simulink subsystem "tire_model"  (R2025b)
settings: Solver=VariableStepAuto  StartTime=0.0  StopTime=10.0  RelTol=1e-3
libraries: vehdynlibtire x3, vehdynlibtirecommon x3
settings Model: Creator=jessi  LastModifiedBy=jessi

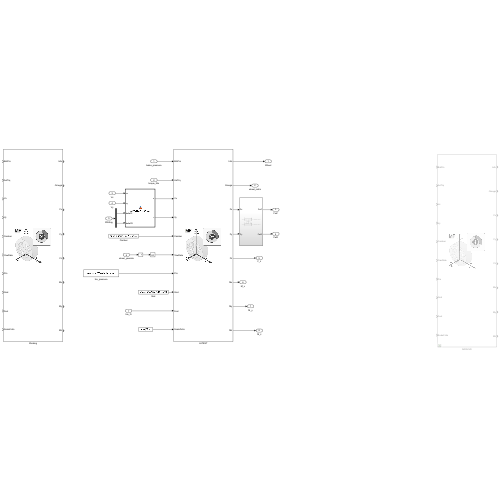
[thumbnail: Simulink's stored preview of the top-level diagram]
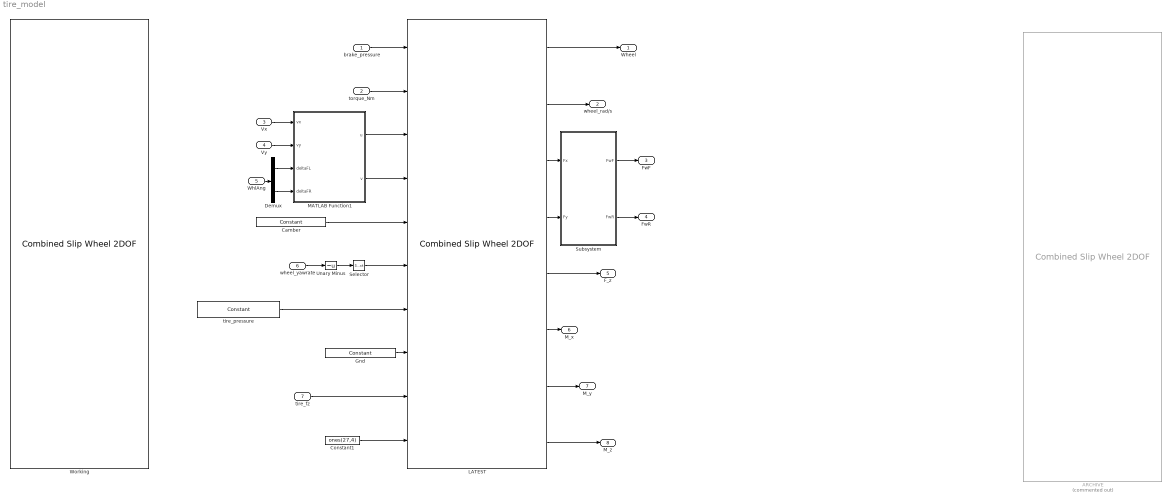
== system tire_model ==
  brake_pressure : Inport  Unit=Pa  PortDimensions=4
  torque_Nm : Inport  Port=2  Unit=N*m  PortDimensions=4
  Vx : Inport  Port=3  Unit=m/s  PortDimensions=4
  Vy : Inport  Port=4  Unit=m/s  PortDimensions=4
  WhlAng : Inport  Port=5
  wheel_yawrate : Inport  Port=6  Unit=rad/s  PortDimensions=1
  tire_fz : Inport  Port=7  Unit=N  PortDimensions=4
  ARCHIVE : vehdynlibtire/Combined Slip Wheel 2DOF  Commented=on  tireType=External file  tireParamSet=C:\Users\jessi\Documents\School\fsae\sim\Hoosier_R25B_B1464_MF.tir  vertType=None  plySteer=off  turnslip=off  BrakeType=Disc  mu_static=.3  mu_kinetic=.2  drum_abore=0.0508  drum_a=0.123  drum_c=0.212  drum_r=0.15  drum_theta1=0  drum_theta2=126  disk_abore=.05  Rm=.177  num_pads=4  brake_p_bpt=[1 11.4736842105263 21.9473684210526 32.4210526315789 42.8947368421053 53.3684210526316 63.8421052631579 74.3157894736842 84.7894736842105 95.2631578947368 105.736842105263 116.210526315789 126.684210526316 137.157894736842 147.631578947368 158.105263157895 168.578947368421 179.052631578947 189.526315789474 200]  brake_n_bpt=[0 52.6315789473684 105.263157894737 157.894736842105 210.526315789474 263.157894736842 315.789473684211 368.421052631579 421.052631578947 473.684210526316 526.315789473684 578.947368421053 631.578947368421 684.210526315789 736.842105263158 789.473684210526 842.105263157895 894.736842105263 947.368421052632 1000]  f_brake_t=[43.4900602404453 42.5056030554862 41.5350898940194 40.5780454442085 39.6340111501808 38.7025443887544 37.7832176914519 36.8756180088306 35.9793460143796 35.0940154454303 34.2192524787115 33.3546951383474 32.4999927342521 31.6548053290159 30.8188032315107 29.991666515561 29.1730845621415 28.362755623661 27.5603864089927 26.765691687993;498.991217495636 487.695866636631 476.560505099801 465.579679307235 454.748127933653 444.060772460445 433.51270824929 423.099196101319 412.81565427025 402.657650900201 392.620896861006 382.701238955775 372.894653477208 363.197240090814 353.605216024701 344.114910546964 334.722759712992 325.425301366216 316.219170376863 307.10109410434;954.492374750826 932.886130217776 911.585920305583 890.581313170261 869.862244717126 849.419000532136 829.242198807128 809.322774193808 789.651962526121 770.221286354971 751.0225412433 732.047782773203 713.289314220164 694.739674852612 676.391628817892 658.238154578366 640.272434863842 622.48784710877 604.877954344734 587.436496520688;1409.99353200602 1378.07639379892 1346.61133551136 1315.58294703329 1284.9763615006 1254.77722860383 1224.97168936497 1195.5463522863 1166.48827078199 1137.78492180974 1109.42418562559 1081.39432659063 1053.68397496312 1026.28210961441 999.178041611083 972.361398609768 945.822110014692 919.550392851325 893.536738312604 867.771898937035;1865.49468926121 1823.26665738007 1781.63675071715 1740.58458089631 1700.09047828407 1660.13545667552 1620.7011799228 1581.76993037878 1543.32457903786 1505.34855726451 1467.82583000789 1430.74087040806 1394.07863570608 1357.82454437621 1321.96445440427 1286.48464264117 1251.37178516554 1216.61293859388 1182.19552228048 1148.10730135338;2320.9958465164 2268.45692096121 2216.66216592293 2165.58621475934 2115.20459506754 2065.49368474721 2016.43067048064 1967.99350847127 1920.16088729373 1872.91219271928 1826.22747439018 1780.08741422549 1734.47329644903 1689.36697913801 1644.75086719747 1600.60788667257 1556.92146031639 1513.67548433643 1470.85430624835 1428.44270376973;2776.49700377159 2713.64718454235 2651.68758112871 2590.58784862237 2530.31871185102 2470.8519128189 2412.16016103848 2354.21708656376 2296.9971955496 2240.47582817405 2184.62911877248 2129.43395804292 2074.86795719199 2020.9094138998 1967.53727999066 1914.73113070398 1862.47113546724 1810.73803007899 1759.51309021622 1708.77810618608;3231.99816102678 3158.8374481235 3086.71299633449 3015.58948248539 2945.43282863449 2876.21014089059 2807.88965159632 2740.44066465625 2673.83350380547 2608.03946362882 2543.03076315477 2478.78050186034 2415.26261793494 2352.4518486616 2290.32369278385 2228.85437473538 2168.02081061809 2107.80057582154 2048.17187418409 1989.11350860242;3687.49931828197 3604.02771170464 3521.73841154027 3440.59111634842 3360.54694541796 3281.56836896228 3203.61914215416 3126.66424274874 3050.66981206134 2975.60309908359 2901.43240753707 2828.12704567777 2755.6572786779 2683.9942834234 2613.11010557704 2542.97761876678 2473.57048576894 2404.8631215641 2336.83065815196 2269.44891101877;4143.00047553716 4049.21797528579 3956.76382674606 3865.59275021144 3775.66106220143 3686.92659703397 3599.34863271199 3512.88782084123 3427.50612031721 3343.16673453836 3259.83405191936 3177.4735894952 3096.05193942085 3015.5367181852 2935.89651837023 2857.10086279818 2779.12016091979 2701.92566730665 2625.48944211983 2549.78431343512;4598.50163279235 4494.40823886693 4391.78924195184 4290.59438407447 4190.77517898491 4092.28482510566 3995.07812326983 3899.11139893372 3804.34242857308 3710.73036999313 3618.23569630166 3526.82013331263 3436.44660016381 3347.079152947 3258.68293116342 3171.22410682959 3084.66983607064 2998.98821304921 2914.1482260877 2830.11971585147;5054.00279004754 4939.59850244808 4826.81465715762 4715.59601793749 4605.88929576838 4497.64305317735 4390.80761382767 4285.3349770262 4181.17873682896 4078.2940054479 3976.63734068395 3876.16667713006 3776.84126090677 3678.62158770879 3581.46934395661 3485.34735086099 ...(+2764 chars)]  NOMPRES=82737.12  PRESMAX=103421  PRESMIN=55158.1  FNOMIN=890.0  FZMAX=3000  FZMIN=100  VXLOW=1  KPUMAX=10  KPUMIN=-1.0  ALPMAX=pi/2  ALPMIN=-pi/2  CAMMAX=0.08726  CAMMIN=-0.08726  LONGVL=11.1  FxRelFreqLwrLim=200*pi  FyRelFreqLwrLim=200*pi  MyRelFreqLwrLim=100*pi  omegao=0  UNLOADED_RADIUS=0.2286  WIDTH=0.1524  RIM_RADIUS=0.127  ASPECT_RATIO=0.67  MASS=9.3  IYY=0.736  br=1e-3  GRAVITY=-9.81  zo=0  zdoto=0  BREFF=0  DREFF=0  FREFF=0  Q_RE0=0  Q_V1=0  Q_V2=0  Q_FZ1=0  Q_FZ2=0  Q_FZ3=0  Q_FCX=0  Q_FCY=0  Q_FCY2=0  PFZ1=0  VERTICAL_STIFFNESS=1  VERTICAL_DAMPING=50  BOTTOM_OFFST=0.01  BOTTOM_STIFF=2000000  Q_CAM1=0  Q_CAM2=0  Q_CAM3=0  Q_FYS1=0  Q_FYS2=0  Q_FYS3=0  LONGITUDINAL_STIFFNESS=183029.97990255515  LATERAL_STIFFNESS=122019.98660170344  PCFX1=6.150634629310016e-19  PCFX2=-0.11842526551903122  PCFX3=0.9999999999999716  PCFY1=6.150634629310016e-19  PCFY2=-0.11842526551903122  PCFY3=0.9999999999999716  Q_RA1=0.671  Q_RA2=0.733  Q_RB1=1.059  Q_RB2=-1.1878  PCX1=1.4779238369371919  PDX1=1.4176795080427544  PDX2=0.07001659216024461  PDX3=4.097157624686553  PEX1=0.24999999999999986  PEX2=-0.4935998299083556  PEX3=0.062308987383295614  PEX4=0.49999999999999994  PKX1=44.40869215364958  PKX2=-0.11467697610242364  PKX3=0.005123300455879327  PHX1=0.00028611316090635194  PHX2=-0.001728319335508632  PVX1=0.004999999999999999  PVX2=0.00477148979863604  PPX1=5.985592437722123e-20  PPX2=-1.4999999999999998  PPX3=-0.45857497477578263  PPX4=-0.43069292241848617  RBX1=7.480599472060266  RBX2=10.358691627632123  RBX3=29.999999999999996  RCX1=1.399999999995603  REX1=-1.1134570691694545  REX2=-0.5558333477828554  RHX1=-9.999999999999997e-07  QSX1=0.0  QSX2=0.5  QSX3=0.05  QSX4=5.0  QSX5=2.0  QSX6=10.0  QSX7=2.0  QSX8=-0.1  QSX9=0.2  QSX10=0.1  QSX11=3.0  QSX12=0  QSX13=0  QSX14=0  PPMX1=0  PCY1=1.42602462123885  PDY1=1.614684806674477  PDY2=-0.25722924030097466  PDY3=7.484237833543449  PEY1=0.24999999999999997  PEY2=0.17282137868029623  PEY3=-0.49999999999981637  PEY4=-18.0131911906531  PEY5=-9.999999999999998  PKY1=-45.05377213726608  PKY2=1.5000000000000002  PKY3=0.9999999999999999  PKY4=1.563548572387517  PKY5=3.062310459473999  PKY6=-4.139177699968599  PKY7=-1.9999999999999998  PHY1=0.002300118354012591  PHY2=-0.0004999941457393199  PVY1=0.06561909162085476  PVY2=-0.057323025837172255  PVY3=-0.7841962281838478  PVY4=-0.4511640295193  PPY1=0.305488175568361  PPY2=0.9999999999971584  PPY3=-0.15059677809127878  PPY4=-6.958531294569729e-28  PPY5=-0.9999999999998861  RBY1=29.999999763033266  RBY2=12.284678148399243  RBY3=9.999999999995652e-07  RBY4=74.99999999999999  RCY1=0.9763806187992715  REY1=0.633343419865921  REY2=0.297623336129197  RHY1=9.999999999999997e-07  RHY2=0.0  RVY1=-0.0009999999999999998  RVY2=-0.001999999999997254  RVY3=-0.049999999999999996  RVY4=1.9999999999999998  RVY5=2.499999999999872  RVY6=-10.881663249213343  QSY1=0.01  QSY2=0.0  QSY3=0.0  QSY4=0.0004  QSY5=0.0  QSY6=0.0  QSY7=0.85  QSY8=0.45  QBZ1=6.523760266884923  QBZ2=-1.0654322141006967  QBZ3=0.0  QBZ4=0.0  QBZ5=-1.0  QBZ6=0  QBZ9=6.716054935778435  QBZ10=0.0  QCZ1=1.1  QDZ1=0.1344522977151938  QDZ2=-0.04833102317146014  QDZ3=0.5  QDZ4=-1.5  QDZ6=0.01667575088116158  QDZ7=-0.026005524615869646  QDZ8=-0.5  QDZ9=0.02  QDZ10=0.0  QDZ11=0.0  QEZ1=-6.042645141020775  QEZ2=5.302859320838443  QEZ3=13.524667353097806  QEZ4=0.17736241081250134  QEZ5=-2.0  QHZ1=0.00824419812657765  QHZ2=0.004999999999999817  QHZ3=0.0  QHZ4=0.0  PPZ1=0.5  PPZ2=0.0  SSZ1=0.0  SSZ2=0.0  SSZ3=0.0  SSZ4=0.0  PDXP1=0.4  PDXP2=0  PDXP3=0  PKYP1=1  PDYP1=0.4  PDYP2=0  PDYP3=0  PDYP4=0  PHYP1=1  PHYP2=0.15  PHYP3=0  PHYP4=-4  PECP1=2.5  PECP2=0.0  QDTP1=10  QCRP1=0.2  QCRP2=0.1  QBRP1=0.1  QDRP1=1  QDRP2=0  aMode=2
  Camber : vehdynlibtirecommon/Constant  const=0  numWheels=4
  Constant1 : Constant  Value=ones(27,4)
  Demux : Demux  Outputs=2
  Gnd : vehdynlibtirecommon/Constant  const=0  numWheels=4
  LATEST : vehdynlibtire/Combined Slip Wheel 2DOF  tireType=External file  tireParamSet=C:\Users\jessi\Documents\School\fsae\sim\heiko_tires_2.tir  vertType=None  plySteer=off  turnslip=off  BrakeType=Disc  mu_static=.3  mu_kinetic=.2  drum_abore=0.0508  drum_a=0.123  drum_c=0.212  drum_r=0.15  drum_theta1=0  drum_theta2=126  disk_abore=.05  Rm=.177  num_pads=4  brake_p_bpt=[1 11.4736842105263 21.9473684210526 32.4210526315789 42.8947368421053 53.3684210526316 63.8421052631579 74.3157894736842 84.7894736842105 95.2631578947368 105.736842105263 116.210526315789 126.684210526316 137.157894736842 147.631578947368 158.105263157895 168.578947368421 179.052631578947 189.526315789474 200]  brake_n_bpt=[0 52.6315789473684 105.263157894737 157.894736842105 210.526315789474 263.157894736842 315.789473684211 368.421052631579 421.052631578947 473.684210526316 526.315789473684 578.947368421053 631.578947368421 684.210526315789 736.842105263158 789.473684210526 842.105263157895 894.736842105263 947.368421052632 1000]  f_brake_t=[43.4900602404453 42.5056030554862 41.5350898940194 40.5780454442085 39.6340111501808 38.7025443887544 37.7832176914519 36.8756180088306 35.9793460143796 35.0940154454303 34.2192524787115 33.3546951383474 32.4999927342521 31.6548053290159 30.8188032315107 29.991666515561 29.1730845621415 28.362755623661 27.5603864089927 26.765691687993;498.991217495636 487.695866636631 476.560505099801 465.579679307235 454.748127933653 444.060772460445 433.51270824929 423.099196101319 412.81565427025 402.657650900201 392.620896861006 382.701238955775 372.894653477208 363.197240090814 353.605216024701 344.114910546964 334.722759712992 325.425301366216 316.219170376863 307.10109410434;954.492374750826 932.886130217776 911.585920305583 890.581313170261 869.862244717126 849.419000532136 829.242198807128 809.322774193808 789.651962526121 770.221286354971 751.0225412433 732.047782773203 713.289314220164 694.739674852612 676.391628817892 658.238154578366 640.272434863842 622.48784710877 604.877954344734 587.436496520688;1409.99353200602 1378.07639379892 1346.61133551136 1315.58294703329 1284.9763615006 1254.77722860383 1224.97168936497 1195.5463522863 1166.48827078199 1137.78492180974 1109.42418562559 1081.39432659063 1053.68397496312 1026.28210961441 999.178041611083 972.361398609768 945.822110014692 919.550392851325 893.536738312604 867.771898937035;1865.49468926121 1823.26665738007 1781.63675071715 1740.58458089631 1700.09047828407 1660.13545667552 1620.7011799228 1581.76993037878 1543.32457903786 1505.34855726451 1467.82583000789 1430.74087040806 1394.07863570608 1357.82454437621 1321.96445440427 1286.48464264117 1251.37178516554 1216.61293859388 1182.19552228048 1148.10730135338;2320.9958465164 2268.45692096121 2216.66216592293 2165.58621475934 2115.20459506754 2065.49368474721 2016.43067048064 1967.99350847127 1920.16088729373 1872.91219271928 1826.22747439018 1780.08741422549 1734.47329644903 1689.36697913801 1644.75086719747 1600.60788667257 1556.92146031639 1513.67548433643 1470.85430624835 1428.44270376973;2776.49700377159 2713.64718454235 2651.68758112871 2590.58784862237 2530.31871185102 2470.8519128189 2412.16016103848 2354.21708656376 2296.9971955496 2240.47582817405 2184.62911877248 2129.43395804292 2074.86795719199 2020.9094138998 1967.53727999066 1914.73113070398 1862.47113546724 1810.73803007899 1759.51309021622 1708.77810618608;3231.99816102678 3158.8374481235 3086.71299633449 3015.58948248539 2945.43282863449 2876.21014089059 2807.88965159632 2740.44066465625 2673.83350380547 2608.03946362882 2543.03076315477 2478.78050186034 2415.26261793494 2352.4518486616 2290.32369278385 2228.85437473538 2168.02081061809 2107.80057582154 2048.17187418409 1989.11350860242;3687.49931828197 3604.02771170464 3521.73841154027 3440.59111634842 3360.54694541796 3281.56836896228 3203.61914215416 3126.66424274874 3050.66981206134 2975.60309908359 2901.43240753707 2828.12704567777 2755.6572786779 2683.9942834234 2613.11010557704 2542.97761876678 2473.57048576894 2404.8631215641 2336.83065815196 2269.44891101877;4143.00047553716 4049.21797528579 3956.76382674606 3865.59275021144 3775.66106220143 3686.92659703397 3599.34863271199 3512.88782084123 3427.50612031721 3343.16673453836 3259.83405191936 3177.4735894952 3096.05193942085 3015.5367181852 2935.89651837023 2857.10086279818 2779.12016091979 2701.92566730665 2625.48944211983 2549.78431343512;4598.50163279235 4494.40823886693 4391.78924195184 4290.59438407447 4190.77517898491 4092.28482510566 3995.07812326983 3899.11139893372 3804.34242857308 3710.73036999313 3618.23569630166 3526.82013331263 3436.44660016381 3347.079152947 3258.68293116342 3171.22410682959 3084.66983607064 2998.98821304921 2914.1482260877 2830.11971585147;5054.00279004754 4939.59850244808 4826.81465715762 4715.59601793749 4605.88929576838 4497.64305317735 4390.80761382767 4285.3349770262 4181.17873682896 4078.2940054479 3976.63734068395 3876.16667713006 3776.84126090677 3678.62158770879 3581.46934395661 3485.34735086099 ...(+2764 chars)]  NOMPRES=82737.12  PRESMAX=103421  PRESMIN=55158.1  FNOMIN=890  FZMAX=2500  FZMIN=100  VXLOW=1  KPUMAX=10  KPUMIN=-1  ALPMAX=1.5708  ALPMIN=-1.5708  CAMMAX=0.08726  CAMMIN=-0.08726  LONGVL=11.1  FxRelFreqLwrLim=200*pi  FyRelFreqLwrLim=200*pi  MyRelFreqLwrLim=100*pi  omegao=0  UNLOADED_RADIUS=0.2286  WIDTH=0.1524  RIM_RADIUS=0.127  ASPECT_RATIO=0.67  MASS=9.3  IYY=0.736  br=1e-3  GRAVITY=-9.81  zo=0  zdoto=0  BREFF=8.386  DREFF=0.25826  FREFF=0.07394  Q_RE0=0.9974  Q_V1=0.00077  Q_V2=0.04667  Q_FZ1=0  Q_FZ2=15.4  Q_FZ3=0  Q_FCX=0  Q_FCY=0  Q_FCY2=0  PFZ1=0.7098  VERTICAL_STIFFNESS=209651  VERTICAL_DAMPING=50  BOTTOM_OFFST=0.01  BOTTOM_STIFF=2000000  Q_CAM1=0  Q_CAM2=0  Q_CAM3=0  Q_FYS1=0  Q_FYS2=0  Q_FYS3=0  LONGITUDINAL_STIFFNESS=180205.884260107  LATERAL_STIFFNESS=120137.256173405  PCFX1=4.99782632605843e-29  PCFX2=0.0455980345994856  PCFX3=1  PCFY1=4.99782632605843e-29  PCFY2=0.0455980345994856  PCFY3=1  Q_RA1=0.671  Q_RA2=0.733  Q_RB1=1.059  Q_RB2=-1.1878  PCX1=1.47792  PDX1=1.41768  PDX2=0.0700166  PDX3=4.09716  PEX1=0.25  PEX2=-0.4936  PEX3=0.062309  PEX4=0.5  PKX1=44.4087  PKX2=-0.114677  PKX3=0.0051233  PHX1=0.000286113  PHX2=-0.00172832  PVX1=0.005  PVX2=0.00477149  PPX1=5.9855924377e-20  PPX2=-1.5  PPX3=-0.458575  PPX4=-0.430693  RBX1=7.4806  RBX2=10.3587  RBX3=30  RCX1=1.4  REX1=-1.11346  REX2=-0.555833  RHX1=-1e-06  QSX1=0  QSX2=0.5  QSX3=0.05  QSX4=5  QSX5=2  QSX6=10  QSX7=2  QSX8=-0.1  QSX9=0.2  QSX10=0.1  QSX11=3  QSX12=0  QSX13=0  QSX14=0  PPMX1=0  PCY1=1.1204  PDY1=1.64222  PDY2=-0.32532  PDY3=8.96121  PEY1=-0.353569  PEY2=0.5  PEY3=0.5  PEY4=-4.334674291e-12  PEY5=-10  PKY1=-58.8756  PKY2=2.6  PKY3=0.82447  PKY4=1.73528  PKY5=0.246779  PKY6=-4.06378  PKY7=-2  PHY1=0.00182546  PHY2=0.000636193  PVY1=0.05  PVY2=-0.0036552  PVY3=0.0983321  PVY4=0.0465855  PPY1=0.569312  PPY2=1  PPY3=-0.151827  PPY4=-1.6963735362e-22  PPY5=-1  RBY1=29.9998  RBY2=12.134  RBY3=9.9999999999e-07  RBY4=75  RCY1=0.965142  REY1=0.61543  REY2=0.174596  RHY1=1e-06  RHY2=0  RVY1=-0.001  RVY2=-0.002  RVY3=-0.05  RVY4=-2  RVY5=2.5  RVY6=-11.3254  QSY1=0.01  QSY2=0  QSY3=0  QSY4=0.0004  QSY5=0  QSY6=0  QSY7=0.85  QSY8=0.45  QBZ1=6.60806  QBZ2=-1.78557  QBZ3=0  QBZ4=0  QBZ5=-1  QBZ6=0  QBZ9=6.54673  QBZ10=0  QCZ1=1.1  QDZ1=0.136052  QDZ2=-0.0673485  QDZ3=0.5  QDZ4=-1.5  QDZ6=0.0171131  QDZ7=-0.028301  QDZ8=-0.5  QDZ9=0.02  QDZ10=0  QDZ11=0  QEZ1=-5.88202  QEZ2=4.83736  QEZ3=13.7151  QEZ4=0.191406  QEZ5=-2  QHZ1=0.00841306  QHZ2=0.005  QHZ3=0  QHZ4=0  PPZ1=0.5  PPZ2=0  SSZ1=0  SSZ2=0  SSZ3=0  SSZ4=0  PDXP1=0.4  PDXP2=0  PDXP3=0  PKYP1=1  PDYP1=0.4  PDYP2=0  PDYP3=0  PDYP4=0  PHYP1=1  PHYP2=0.15  PHYP3=0  PHYP4=-4  PECP1=0.5  PECP2=0  QDTP1=10  QCRP1=0.2  QCRP2=0.1  QBRP1=0.1  QDRP1=1  QDRP2=0  aMode=2
  MATLAB Function1 : MATLAB Function  TreatAsAtomicUnit=on
  Selector : Selector  InputPortWidth=1  IndexOptions=Index vector (dialog)  Indices=[1 1 1 1]  OutputSizes=1
  Subsystem : Subsystem
  Unary Minus : UnaryMinus
  Working : vehdynlibtire/Combined Slip Wheel 2DOF  tireType=External file  vertType=None  plySteer=off  turnslip=off  BrakeType=Disc  mu_static=.3  mu_kinetic=.2  drum_abore=0.0508  drum_a=0.123  drum_c=0.212  drum_r=0.15  drum_theta1=0  drum_theta2=126  disk_abore=.05  Rm=.177  num_pads=4  brake_p_bpt=[1 11.4736842105263 21.9473684210526 32.4210526315789 42.8947368421053 53.3684210526316 63.8421052631579 74.3157894736842 84.7894736842105 95.2631578947368 105.736842105263 116.210526315789 126.684210526316 137.157894736842 147.631578947368 158.105263157895 168.578947368421 179.052631578947 189.526315789474 200]  brake_n_bpt=[0 52.6315789473684 105.263157894737 157.894736842105 210.526315789474 263.157894736842 315.789473684211 368.421052631579 421.052631578947 473.684210526316 526.315789473684 578.947368421053 631.578947368421 684.210526315789 736.842105263158 789.473684210526 842.105263157895 894.736842105263 947.368421052632 1000]  f_brake_t=[43.4900602404453 42.5056030554862 41.5350898940194 40.5780454442085 39.6340111501808 38.7025443887544 37.7832176914519 36.8756180088306 35.9793460143796 35.0940154454303 34.2192524787115 33.3546951383474 32.4999927342521 31.6548053290159 30.8188032315107 29.991666515561 29.1730845621415 28.362755623661 27.5603864089927 26.765691687993;498.991217495636 487.695866636631 476.560505099801 465.579679307235 454.748127933653 444.060772460445 433.51270824929 423.099196101319 412.81565427025 402.657650900201 392.620896861006 382.701238955775 372.894653477208 363.197240090814 353.605216024701 344.114910546964 334.722759712992 325.425301366216 316.219170376863 307.10109410434;954.492374750826 932.886130217776 911.585920305583 890.581313170261 869.862244717126 849.419000532136 829.242198807128 809.322774193808 789.651962526121 770.221286354971 751.0225412433 732.047782773203 713.289314220164 694.739674852612 676.391628817892 658.238154578366 640.272434863842 622.48784710877 604.877954344734 587.436496520688;1409.99353200602 1378.07639379892 1346.61133551136 1315.58294703329 1284.9763615006 1254.77722860383 1224.97168936497 1195.5463522863 1166.48827078199 1137.78492180974 1109.42418562559 1081.39432659063 1053.68397496312 1026.28210961441 999.178041611083 972.361398609768 945.822110014692 919.550392851325 893.536738312604 867.771898937035;1865.49468926121 1823.26665738007 1781.63675071715 1740.58458089631 1700.09047828407 1660.13545667552 1620.7011799228 1581.76993037878 1543.32457903786 1505.34855726451 1467.82583000789 1430.74087040806 1394.07863570608 1357.82454437621 1321.96445440427 1286.48464264117 1251.37178516554 1216.61293859388 1182.19552228048 1148.10730135338;2320.9958465164 2268.45692096121 2216.66216592293 2165.58621475934 2115.20459506754 2065.49368474721 2016.43067048064 1967.99350847127 1920.16088729373 1872.91219271928 1826.22747439018 1780.08741422549 1734.47329644903 1689.36697913801 1644.75086719747 1600.60788667257 1556.92146031639 1513.67548433643 1470.85430624835 1428.44270376973;2776.49700377159 2713.64718454235 2651.68758112871 2590.58784862237 2530.31871185102 2470.8519128189 2412.16016103848 2354.21708656376 2296.9971955496 2240.47582817405 2184.62911877248 2129.43395804292 2074.86795719199 2020.9094138998 1967.53727999066 1914.73113070398 1862.47113546724 1810.73803007899 1759.51309021622 1708.77810618608;3231.99816102678 3158.8374481235 3086.71299633449 3015.58948248539 2945.43282863449 2876.21014089059 2807.88965159632 2740.44066465625 2673.83350380547 2608.03946362882 2543.03076315477 2478.78050186034 2415.26261793494 2352.4518486616 2290.32369278385 2228.85437473538 2168.02081061809 2107.80057582154 2048.17187418409 1989.11350860242;3687.49931828197 3604.02771170464 3521.73841154027 3440.59111634842 3360.54694541796 3281.56836896228 3203.61914215416 3126.66424274874 3050.66981206134 2975.60309908359 2901.43240753707 2828.12704567777 2755.6572786779 2683.9942834234 2613.11010557704 2542.97761876678 2473.57048576894 2404.8631215641 2336.83065815196 2269.44891101877;4143.00047553716 4049.21797528579 3956.76382674606 3865.59275021144 3775.66106220143 3686.92659703397 3599.34863271199 3512.88782084123 3427.50612031721 3343.16673453836 3259.83405191936 3177.4735894952 3096.05193942085 3015.5367181852 2935.89651837023 2857.10086279818 2779.12016091979 2701.92566730665 2625.48944211983 2549.78431343512;4598.50163279235 4494.40823886693 4391.78924195184 4290.59438407447 4190.77517898491 4092.28482510566 3995.07812326983 3899.11139893372 3804.34242857308 3710.73036999313 3618.23569630166 3526.82013331263 3436.44660016381 3347.079152947 3258.68293116342 3171.22410682959 3084.66983607064 2998.98821304921 2914.1482260877 2830.11971585147;5054.00279004754 4939.59850244808 4826.81465715762 4715.59601793749 4605.88929576838 4497.64305317735 4390.80761382767 4285.3349770262 4181.17873682896 4078.2940054479 3976.63734068395 3876.16667713006 3776.84126090677 3678.62158770879 3581.46934395661 3485.34735086099 ...(+2764 chars)]  NOMPRES=82737.12  PRESMAX=103421  PRESMIN=55158.1  FNOMIN=890.0  FZMAX=5000  FZMIN=100  VXLOW=1  KPUMAX=10  KPUMIN=-1.0  ALPMAX=pi/2  ALPMIN=-pi/2  CAMMAX=0.08726  CAMMIN=-0.08726  LONGVL=11.1  FxRelFreqLwrLim=200*pi  FyRelFreqLwrLim=200*pi  MyRelFreqLwrLim=100*pi  omegao=0  UNLOADED_RADIUS=0.2286  WIDTH=0.1524  RIM_RADIUS=0.127  ASPECT_RATIO=0.67  MASS=9.3  IYY=0.736  br=1e-3  GRAVITY=-9.81  zo=0  zdoto=0  BREFF=8.386  DREFF=0.25826  FREFF=0.07394  Q_RE0=0.9974  Q_V1=0.00077  Q_V2=0.04667  Q_FZ1=0  Q_FZ2=15.4  Q_FZ3=0  Q_FCX=0  Q_FCY=0  Q_FCY2=0  PFZ1=0.7098  VERTICAL_STIFFNESS=209651  VERTICAL_DAMPING=50  BOTTOM_OFFST=0.01  BOTTOM_STIFF=2000000  Q_CAM1=0  Q_CAM2=0  Q_CAM3=0  Q_FYS1=0  Q_FYS2=0  Q_FYS3=0  LONGITUDINAL_STIFFNESS=358066  LATERAL_STIFFNESS=102673  PCFX1=0.17504  PCFX2=0  PCFX3=0  PCFY1=0.16365  PCFY2=0  PCFY3=0.24993  Q_RA1=0.671  Q_RA2=0.733  Q_RB1=1.059  Q_RB2=-1.1878  PCX1=1.4759319652841167  PDX1=2.1796047139413703  PDX2=-0.4291518578855814  PDX3=9.999999999999998  PEX1=0.24999999999999992  PEX2=0.4999999999503354  PEX3=-0.19999999998013418  PEX4=0.49999999999999994  PKX1=44.486722871854106  PKX2=0.7120674645715347  PKX3=0.05499344672791521  PHX1=0.00028868605457366223  PHX2=0.0019999999988281974  PVX1=0.004999999999999999  PVX2=-0.004999999999999571  PPX1=2.4205061531330237e-17  PPX2=-0.9573016482413841  PPX3=-0.44725115013003364  PPX4=-1.0829178486140199  RBX1=7.492442914324831  RBX2=10.346089331771397  RBX3=29.999999999999996  RCX1=1.3999999999999924  REX1=-1.157802528712476  REX2=0.9999999999999999  RHX1=-9.999999999999997e-07  QSX1=0.0  QSX2=0.5  QSX3=0.05  QSX4=5.0  QSX5=2.0  QSX6=10.0  QSX7=2.0  QSX8=-0.1  QSX9=0.2  QSX10=0.1  QSX11=3.0  QSX12=0  QSX13=0  QSX14=0  PPMX1=0  PCY1=1.4260605641217314  PDY1=2.4841487233120225  PDY2=-0.1876440219775705  PDY3=7.508428290647241  PEY1=0.24999999999999997  PEY2=-0.499999999999991  PEY3=-0.49999999999981753  PEY4=-18.269893351294126  PEY5=9.999999999999998  PKY1=-45.05302401059848  PKY2=2.1781682283379564  PKY3=-0.17604712854342697  PKY4=1.9426288921522195  PKY5=4.999999999999999  PKY6=-4.17394673832909  PKY7=-1.7192793969581321  PHY1=0.0023001682759390277  PHY2=0.0031347378176419653  PVY1=0.06560934751893403  PVY2=0.11060727790094066  PVY3=-0.7870245501487243  PVY4=1.9999999990891213  PPY1=0.15987950056064024  PPY2=0.8091878858639612  PPY3=-0.0679339736908627  PPY4=-0.3106544629486843  PPY5=-0.9999999999987371  RBY1=23.942508490286457  RBY2=10.659317359995574  RBY3=7.459484998984083e-07  RBY4=-74.99999999999963  RCY1=0.9838718951518215  REY1=0.571655288653177  REY2=0.6687626858266051  RHY1=9.99998578319522e-07  RHY2=0.0  RVY1=0.0009999999999997134  RVY2=0.001999999999999887  RVY3=-0.049999999999999996  RVY4=-1.9999999999999998  RVY5=2.4999447302580524  RVY6=9.5344602632312  QSY1=0.01  QSY2=0.0  QSY3=0.0  QSY4=0.0004  QSY5=0.0  QSY6=0.0  QSY7=0.85  QSY8=0.45  QBZ1=10.0  QBZ2=-2.0  QBZ3=0.0  QBZ4=0.0  QBZ5=-1.0  QBZ6=0  QBZ9=15.0  QBZ10=0.0  QCZ1=1.1  QDZ1=0.12  QDZ2=-0.02  QDZ3=0.5  QDZ4=-1.5  QDZ6=-0.01  QDZ7=0.01  QDZ8=-0.5  QDZ9=0.02  QDZ10=0.0  QDZ11=0.0  QEZ1=-1.5  QEZ2=-0.5  QEZ3=0.0  QEZ4=0.2  QEZ5=-2.0  QHZ1=0.005  QHZ2=0.002  QHZ3=0.0  QHZ4=0.0  PPZ1=0.5  PPZ2=0.0  SSZ1=0.0  SSZ2=0.0  SSZ3=0.0  SSZ4=0.0  PDXP1=0.4  PDXP2=0  PDXP3=0  PKYP1=1  PDYP1=0.4  PDYP2=0  PDYP3=0  PDYP4=0  PHYP1=1  PHYP2=0.15  PHYP3=0  PHYP4=-4  PECP1=2.5  PECP2=0.0  QDTP1=10  QCRP1=0.2  QCRP2=0.1  QBRP1=0.1  QDRP1=1  QDRP2=0  aMode=2
  tire_pressure : vehdynlibtirecommon/Constant  const=2.4e5*1.1  numWheels=4
  Wheel : Outport
  wheel_rad/s : Outport  Port=2  Unit=rad/s  PortDimensions=4
  FwF : Outport  Port=3  Unit=N  PortDimensions=[2 2]
  FwR : Outport  Port=4  PortDimensions=[2 2]
  F_z : Outport  Port=5
  M_x : Outport  Port=6
  M_y : Outport  Port=7
  M_z : Outport  Port=8
  wires:
  WhlAng/1 -> Demux/1
  Subsystem/1(FwF) -> FwF/1
  Subsystem/2(FwR) -> FwR/1
  Vx/1 -> MATLAB Function1/1(vx)
  Vy/1 -> MATLAB Function1/2(vy)
  Demux/1 -> MATLAB Function1/3(deltaFL)
  Demux/2 -> MATLAB Function1/4(deltaFR)
  wheel_yawrate/1 -> Unary Minus/1
  Unary Minus/1 -> Selector/1
  tire_fz/1 -> LATEST/9
  LATEST/4 -> Subsystem/2(Fy)
  Gnd/1 -> LATEST/8
  Camber/1 -> LATEST/5
  tire_pressure/1 -> LATEST/7
  torque_Nm/1 -> LATEST/2
  LATEST/2 -> wheel_rad/s/1
  MATLAB Function1/1(u) -> LATEST/3
  LATEST/5 -> F_z/1
  LATEST/6 -> M_x/1
  LATEST/7 -> M_y/1
  LATEST/8 -> M_z/1
  Selector/1 -> LATEST/6
  Constant1/1 -> LATEST/10
  brake_pressure/1 -> LATEST/1
  LATEST/3 -> Subsystem/1(Fx)
  MATLAB Function1/2(v) -> LATEST/4
  LATEST/1 -> Wheel/1

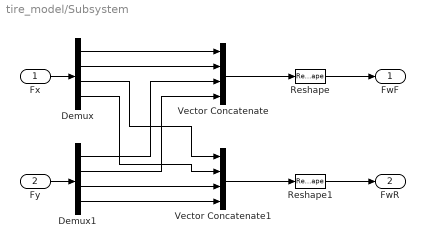
== system tire_model/Subsystem ==
  Fx : Inport
  Fy : Inport  Port=2
  Demux : Demux
  Demux1 : Demux
  Reshape : Reshape  OutputDimensionality=Customize  OutputDimensions=[2,2]
  Reshape1 : Reshape  OutputDimensionality=Customize  OutputDimensions=[2,2]
  Vector Concatenate : Concatenate  NumInputs=4
  Vector Concatenate1 : Concatenate  NumInputs=4
  FwF : Outport
  FwR : Outport  Port=2
  wires:
  Reshape/1 -> FwF/1
  Demux1/2 -> Vector Concatenate/4
  Fx/1 -> Demux/1
  Demux1/4 -> Vector Concatenate1/4
  Demux1/3 -> Vector Concatenate1/3
  Demux1/1 -> Vector Concatenate/3
  Demux/3 -> Vector Concatenate1/1
  Fy/1 -> Demux1/1
  Demux/4 -> Vector Concatenate1/2
  Demux/1 -> Vector Concatenate/1
  Vector Concatenate/1 -> Reshape/1
  Demux/2 -> Vector Concatenate/2
  Vector Concatenate1/1 -> Reshape1/1
  Reshape1/1 -> FwR/1

== matlab function tire_model/MATLAB Function1 ==
  data: vx input; u output; vy input; deltaFL input; deltaFR input; v output
function [u, v] = vehToTireFrontSteer(vx, vy, deltaFL, deltaFR)
%#codegen
u = zeros(4,1);
v = zeros(4,1);

vx = reshape(vx,4,1);
vy = reshape(vy,4,1);

delta = [deltaFL; deltaFR; 0; 0];   % 4×1

cd = cos(delta);
sd = sin(delta);

u =  vx.*cd + vy.*sd;   % 4×1
v = -vx.*sd + vy.*cd;   % 4×1
end
